simulink model "quadSimulink"  (R2017a)
settings: Solver=VariableStepAuto  StartTime=0.0  StopTime=30.0  RelTol=1e-3
undefined symbols (not defined in the file): dx0, dy0, dz0, p0, phi0, psi0, q0, r0, theta0, x0, y0, z0
settings Model: Creator=gianl  LastModifiedBy=gianl

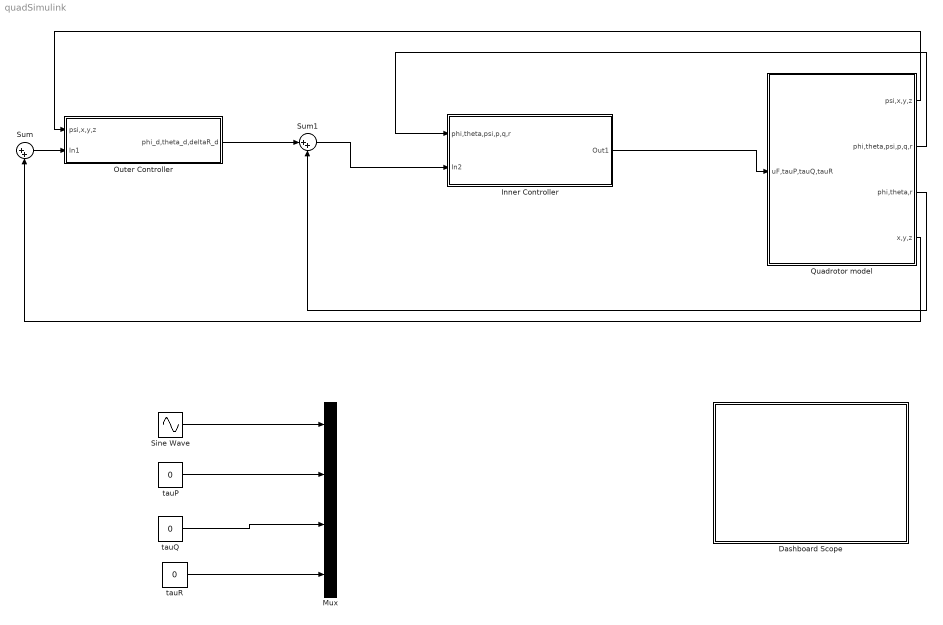
== system quadSimulink ==
  Dashboard Scope : Subsystem  DialogController=hmiCreateDDGDialog  IsWebBlock=on  mask(MWDashboardBlock){webBlockId=5c95f074-7ca7-4b97-9ad1-08e7da2f8987, webBlockType=sdiscope, ShowInitialText=on, HMISrcModelName=quadSimulink}
      mask prompts: webBlockId "WebBlock Id"; webBlockType "WebBlock Type"; HMISrcModelName "Source Model"
      mask help: SimulinkHMI:dialogs:HMIScopeDialogDesc
      mask Help: helpview([docroot '/mapfiles/simulink.map'], 'hmi_scope')
      mask Display:
      | if strcmp(get_param(bdroot(gcb),'BlockDiagramType'), 'library')
      |     image([(matlabroot) '/toolbox/simulink/hmi/icons/DashboardScope.png']);
      | end
  "Inner Controller " : Subsystem
  Mux : Mux
  "Outer Controller " : Subsystem
  "Quadrotor model " : Subsystem
  Sine Wave : Sin  Amplitude=8  SampleTime=0
  Sum : Sum  Inputs=|++
  Sum1 : Sum  Inputs=|++
  tauP : Constant  Value=0
  tauQ : Constant  Value=0
  tauR : Constant  Value=0
  wires:
  "Outer Controller "/1("phi_d,theta_d,deltaR_d ") -> Sum1/1
  Sum/1 -> "Outer Controller "/2(In1)
  "Quadrotor model "/4(x,y,z) -> Sum/2
  "Quadrotor model "/3("phi,theta,r ") -> Sum1/2
  "Quadrotor model "/1("psi,x,y,z ") -> "Outer Controller "/1(psi,x,y,z)
  "Quadrotor model "/2("phi,theta,psi,p,q,r ") -> "Inner Controller "/1(phi,theta,psi,p,q,r)
  Sum1/1 -> "Inner Controller "/2(In2)
  Sine Wave/1 -> Mux/1
  tauP/1 -> Mux/2
  tauR/1 -> Mux/4
  "Inner Controller "/1(Out1) -> "Quadrotor model "/1(uF,tauP,tauQ,tauR)
  tauQ/1 -> Mux/3

== system quadSimulink/Dashboard Scope ==

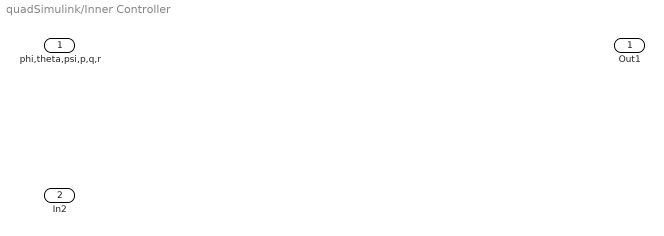
== system quadSimulink/Inner Controller  ==
  phi,theta,psi,p,q,r : Inport
  In2 : Inport  Port=2
  Out1 : Outport

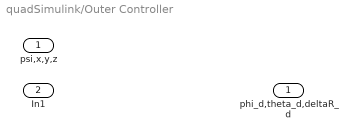
== system quadSimulink/Outer Controller  ==
  psi,x,y,z : Inport
  In1 : Inport  Port=2
  "phi_d,theta_d,deltaR_d " : Outport

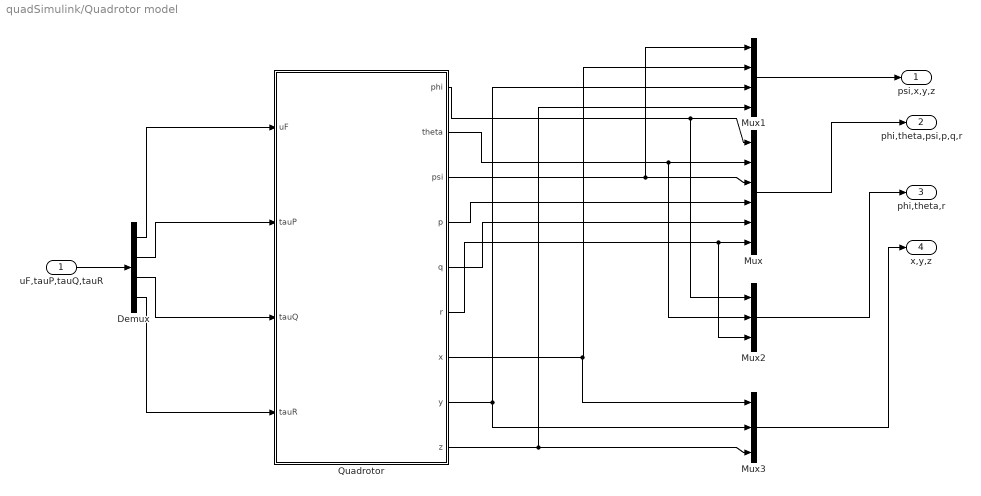
== system quadSimulink/Quadrotor model  ==
  uF,tauP,tauQ,tauR : Inport
  Demux : Demux
  Mux : Mux  Inputs=6
  Mux1 : Mux
  Mux2 : Mux  Inputs=3
  Mux3 : Mux  Inputs=3
  "Quadrotor " : Subsystem
  "psi,x,y,z " : Outport
  "phi,theta,psi,p,q,r " : Outport  Port=2
  "phi,theta,r " : Outport  Port=3
  x,y,z : Outport  Port=4
  wires:
  uF,tauP,tauQ,tauR/1 -> Demux/1
  Mux1/1 -> "psi,x,y,z "/1
  Mux/1 -> "phi,theta,psi,p,q,r "/1
  Mux2/1 -> "phi,theta,r "/1
  Mux3/1 -> x,y,z/1
  "Quadrotor "/1(phi) -> Mux2/1, Mux/1
  "Quadrotor "/2(theta) -> Mux2/2, Mux/2
  "Quadrotor "/3(psi) -> Mux/3, Mux1/1
  "Quadrotor "/4(p) -> Mux/4
  "Quadrotor "/5(q) -> Mux/5
  "Quadrotor "/6(r) -> Mux/6, Mux2/3
  "Quadrotor "/7(x) -> Mux3/1, Mux1/2
  "Quadrotor "/8(y) -> Mux1/3, Mux3/2
  "Quadrotor "/9(z) -> Mux1/4, Mux3/3
  Demux/1 -> "Quadrotor "/1(uF)
  Demux/2 -> "Quadrotor "/2(tauP)
  Demux/3 -> "Quadrotor "/3(tauQ)
  Demux/4 -> "Quadrotor "/4(tauR)

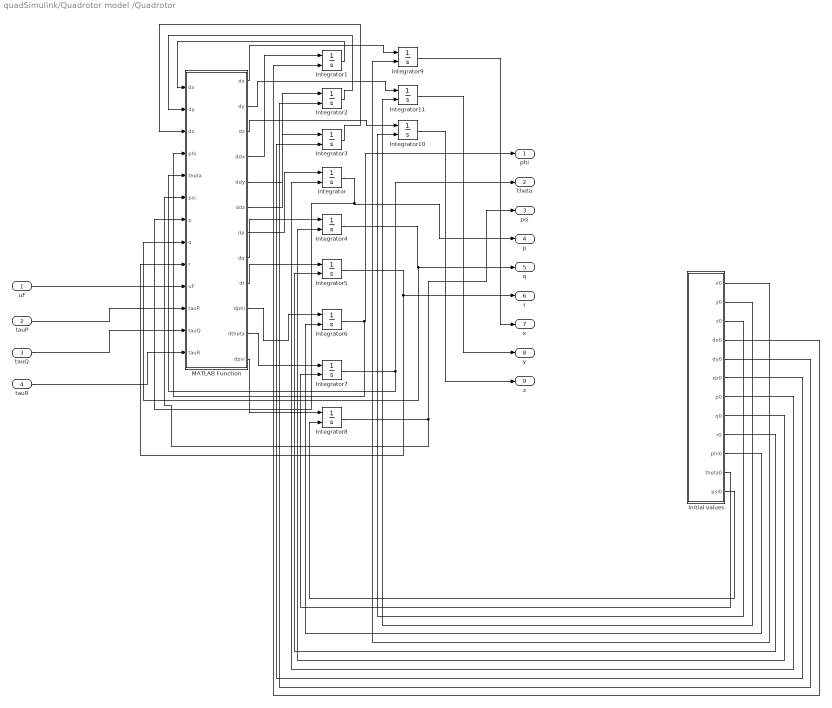
== system quadSimulink/Quadrotor model /Quadrotor  ==
  uF : Inport
  tauP : Inport  Port=2
  tauQ : Inport  Port=3
  tauR : Inport  Port=4
  "Initial values " : Subsystem
  Integrator{,1..11} (12 alike) : Integrator  InitialConditionSource=external
  MATLAB Function : MATLAB Function  TreatAsAtomicUnit=on
  phi : Outport
  theta : Outport  Port=2
  psi : Outport  Port=3
  p : Outport  Port=4
  q : Outport  Port=5
  r : Outport  Port=6
  x : Outport  Port=7
  y : Outport  Port=8
  z : Outport  Port=9
  wires:
  uF/1 -> MATLAB Function/10(uF)
  tauP/1 -> MATLAB Function/11(tauP)
  tauQ/1 -> MATLAB Function/12(tauQ)
  tauR/1 -> MATLAB Function/13(tauR)
  MATLAB Function/12(dpsi) -> Integrator8/1
  Integrator8/1 -> MATLAB Function/6(psi), psi/1
  MATLAB Function/11(dtheta) -> Integrator7/1
  Integrator7/1 -> MATLAB Function/5(theta), theta/1
  MATLAB Function/10(dphi) -> Integrator6/1
  Integrator6/1 -> MATLAB Function/4(phi), phi/1
  MATLAB Function/9(dr) -> Integrator5/1
  Integrator5/1 -> MATLAB Function/9(r), r/1
  MATLAB Function/8(dq) -> Integrator4/1
  Integrator4/1 -> MATLAB Function/8(q), q/1
  MATLAB Function/7(dp) -> Integrator/1
  Integrator/1 -> MATLAB Function/7(p), p/1
  MATLAB Function/6(ddz) -> Integrator3/1
  MATLAB Function/5(ddy) -> Integrator2/1
  MATLAB Function/4(ddx) -> Integrator1/1
  Integrator3/1 -> MATLAB Function/3("dz ")
  Integrator2/1 -> MATLAB Function/2("dy ")
  Integrator1/1 -> MATLAB Function/1("dx ")
  Integrator9/1 -> x/1
  Integrator11/1 -> y/1
  Integrator10/1 -> z/1
  "Initial values "/1(x0) -> Integrator9/2
  "Initial values "/2(y0) -> Integrator11/2
  "Initial values "/3(z0) -> Integrator10/2
  "Initial values "/4(dx0) -> Integrator1/2
  "Initial values "/5(dy0) -> Integrator2/2
  "Initial values "/6(dz0) -> Integrator3/2
  "Initial values "/7(p0) -> Integrator/2
  "Initial values "/8(q0) -> Integrator4/2
  "Initial values "/9(r0) -> Integrator5/2
  "Initial values "/10(phi0) -> Integrator6/2
  "Initial values "/11(theta0) -> Integrator7/2
  "Initial values "/12(psi0) -> Integrator8/2
  MATLAB Function/1(dx) -> Integrator9/1
  MATLAB Function/2(dy) -> Integrator11/1
  MATLAB Function/3(dz) -> Integrator10/1

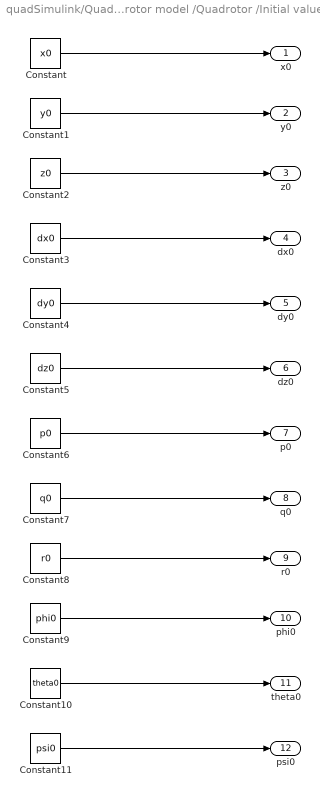
== system quadSimulink/Quadrotor model /Quadrotor /Initial values  ==
  Constant : Constant  Value=x0
  Constant1 : Constant  Value=y0
  Constant10 : Constant  Value=theta0
  Constant11 : Constant  Value=psi0
  Constant2 : Constant  Value=z0
  Constant3 : Constant  Value=dx0
  Constant4 : Constant  Value=dy0
  Constant5 : Constant  Value=dz0
  Constant6 : Constant  Value=p0
  Constant7 : Constant  Value=q0
  Constant8 : Constant  Value=r0
  Constant9 : Constant  Value=phi0
  x0 : Outport
  y0 : Outport  Port=2
  z0 : Outport  Port=3
  dx0 : Outport  Port=4
  dy0 : Outport  Port=5
  dz0 : Outport  Port=6
  p0 : Outport  Port=7
  q0 : Outport  Port=8
  r0 : Outport  Port=9
  phi0 : Outport  Port=10
  theta0 : Outport  Port=11
  psi0 : Outport  Port=12
  wires:
  Constant/1 -> x0/1
  Constant1/1 -> y0/1
  Constant2/1 -> z0/1
  Constant3/1 -> dx0/1
  Constant4/1 -> dy0/1
  Constant5/1 -> dz0/1
  Constant6/1 -> p0/1
  Constant7/1 -> q0/1
  Constant8/1 -> r0/1
  Constant9/1 -> phi0/1
  Constant10/1 -> theta0/1
  Constant11/1 -> psi0/1

== matlab function quadSimulink/Quadrotor model /Quadrotor /MATLAB Function ==
  data: dx output; dy output; dz output; dx input; dy input; dz input; phi input; theta input; psi input; p input; q input; r input; uF input; ddx output; tauP input; tauQ input; tauR input; ddy output; ddz output; dp output; dq output; dr output; dphi output; dtheta output; dpsi output
function [dx,dy,dz,ddx,ddy,ddz,dp,dq,dr,dphi,dtheta,dpsi] = fcn(dx, dy, dz, phi, theta, psi, p, q, r, uF, tauP, tauQ, tauR)
    
    g = 9.81;
    m = 0.5;
    %l = 0.255;
    %d = 2.4*10^(-3);
    
    kt = 1;
    kr = 1;

    Ixx = 5.9*10^(-3);
    Iyy = 5.9*10^(-3);
    Izz = 1.16*10^(-3);

    
    ddx = (1/m)*((cos(phi)*cos(psi)*sin(theta) + sin(phi)*sin(psi))*uF - kt*dx);
    
    ddy = (1/m)*((cos(phi)*sin(theta)*sin(psi) - cos(psi)*sin(phi))*uF - kt*dy);
    
    ddz = (1/m)*((cos(theta)*cos(phi))*uF - m*g - kt*dz);
    
    dp = (1/Ixx)*(-kr*p - q*r*(Izz - Iyy) + tauP);
    
    dq = (1/Iyy)*(-kr*q - p*r*(Ixx - Izz) + tauQ);
    
    dr = (1/Izz)*(-kr*r - p*q*(Iyy - Ixx) + tauR);
    
    dphi = p + q*sin(phi)*tan(phi) + r*cos(phi)*tan(theta);
    
    dtheta = q*cos(phi) - r*sin(phi);
    
    dpsi = (1/cos(theta))*(q*sin(phi) + r*cos(phi));
